simulink model "sfcndemo_csfunc"  (Simulink 6.0)
settings: Solver=ode3  SolverMode=SingleTasking  StartTime=0.0  StopTime=10  FixedStep=.01  MaxStep=0.01  RelTol=1e-3  AbsTol=1e-6
settings Model: Creator=The MathWorks Inc.  LastModifiedBy=batserve  ExtModeTrigMode=oneshot  ExtModeArmWhenConnect=off  ExtModeAutoUpdateStatusClock=off
settings DataIOCC: ExternalInput=[]  InitialState=[]  LimitDataPoints=off
settings OptimizationCC: BooleanDataType=off
settings DebuggingCC: CheckExecutionContextPreStartOutputMsg=on  CheckExecutionContextRuntimeOutputMsg=on  SolverPrmCheckMsg=none  InheritedTsInSrcMsg=none
settings HardwareCC: TargetUnknown=on

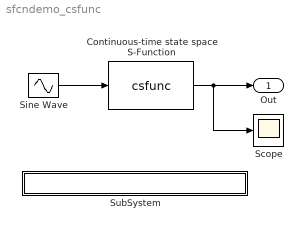
== system sfcndemo_csfunc ==
  Continuous-time state space S-Function : S-Function  FunctionName=csfunc
      mask Type: S-function: csfunc
      mask Description: This is a S-function that does the continuous state space system.
      mask Display: disp('x'' = A*X + B*U\n Y = C*X + D*U ');
  Scope : Scope
      settings: TimeRange=10  YMin=-200  YMax=500
  Sine Wave : Sin  Amplitude=[1 2]  SampleTime=0
  SubSystem : Subsystem  PropExecContextAcrossSSBoundary=on
      settings: OpenFcn=edit(fullfile(matlabroot,'simulink','src','csfunc.c'))
      mask Display: disp('matlabroot\simulink\src\csfunc.c');
  Out : Outport  InitialOutput=0
  wires:
  Sine Wave/1 -> Continuous-time state space S-Function/1
  Continuous-time state space S-Function/1 -> Out/1, Scope/1

== system sfcndemo_csfunc/SubSystem ==
